simulink model "modelo_function"  (R2017a)
settings: Solver=VariableStepAuto  StartTime=0.0  StopTime=20.0  MaxStep=1e-4  RelTol=1e-3
values from neighbouring files (symbols this model uses):
  a = -subs(y_lin, [y yd u], [0 1 0])    [linearization.m]    (also in preConfig.m = 0.97)
  b = -subs(y_lin, [y yd u], [1 0 0])    [linearization.m]    (also in preConfig.m = 6.4)
  c = .15    (= 0.15)    [preConfig.m]
  g = 9.8    [preConfig.m]
  m = 0.12    [preConfig.m]
  N = 4    [preConfig.m]
settings Model: Creator=Herculano  LastModifiedBy=Herculano

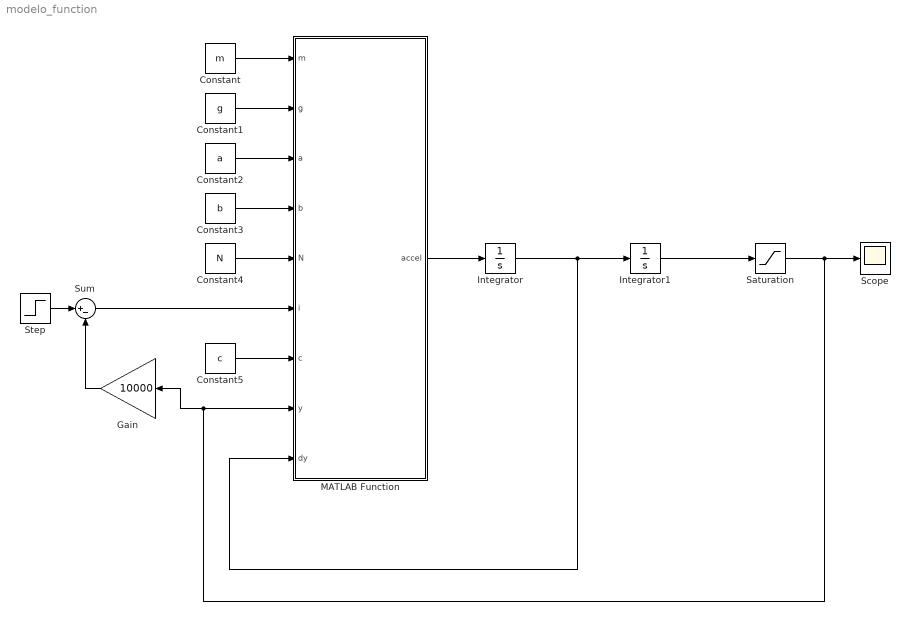
== system modelo_function ==
  Constant : Constant  Value=m
  Constant1 : Constant  Value=g
  Constant2 : Constant  Value=a
  Constant3 : Constant  Value=b
  Constant4 : Constant  Value=N
  Constant5 : Constant  Value=c
  Gain : Gain  Gain=10000
  Integrator : Integrator
  Integrator1 : Integrator
  MATLAB Function : MATLAB Function  TreatAsAtomicUnit=on
  Saturation : Saturate  UpperLimit=10000  LowerLimit=0
  Scope : Scope
  Step : Step  Time=0  After=15000  SampleTime=0
  Sum : Sum  Inputs=|+-
  wires:
  Constant/1 -> MATLAB Function/1(m)
  Constant1/1 -> MATLAB Function/2(g)
  Constant2/1 -> MATLAB Function/3(a)
  Constant3/1 -> MATLAB Function/4(b)
  Constant4/1 -> MATLAB Function/5(N)
  Constant5/1 -> MATLAB Function/7(c)
  MATLAB Function/1(accel) -> Integrator/1
  Integrator/1 -> MATLAB Function/9(dy), Integrator1/1
  Integrator1/1 -> Saturation/1
  Saturation/1 -> Scope/1, MATLAB Function/8(y), Gain/1
  Step/1 -> Sum/1
  Sum/1 -> MATLAB Function/6(i)
  Gain/1 -> Sum/2

== matlab function modelo_function/MATLAB Function ==
  data: m input; g input; accel output; a input; b input; N input; i input; c input; y input; dy input
function accel = fcn(m,g,a,b,N,i,c,y,dy)
    accel = i/(m*a*(y+b)^N) - g - c * dy/m;
